simulink library "NCS_Library"  (R2019a)
settings: Solver=VariableStepAuto  StartTime=0.0  StopTime=10.0  RelTol=1e-3
values from neighbouring files (symbols this model uses):
  A = 10    [Parameter.m]
  band = 100000000    [Parameter.m]
  BER = 0    [Parameter.m]
  c = 5000000    [Parameter.m]
  c1 = 4.33    [Parameter.m]
  c2 = 3.16    [Parameter.m]
  CAN2EthernetDelay = 0.000    (= 0)    [Parameter.m]
  cR = 1.5*10^-3    (= 0.0015)    [Parameter.m]
  cw = (cwE * 2 + cwM * (nW_ges-2))/nW_ges    (= 0.1475)    [Parameter.m]
  cwE = 0.35    [Parameter.m]
  cwM = 0.08    [Parameter.m]
  Cycle_Controller = 0    [Parameter.m]
  CyclePLC = 24/1000    (= 0.024)    [Parameter.m]
  d = 800000    [Parameter.m]
  Dr = 0.92    [Parameter.m]
  Ethernet2CANDelay = 0.005    [Parameter.m]
  F_konst = 70892    [Parameter.m]
  FA = 100000    [Parameter.m]
  FB_WB_max = 10000    [Parameter.m]
  FBel_an = iG*nG*F_KZmax*nBan*R_mR/(Dr/2)    (= 28197.4297239)    [Parameter.m]
  FBel_frei = iG*nG*F_KZmax*nBfrei*R_mW/(Dr/2)    (= 29270.6882948)    [Parameter.m]
  Fmaxdyn = 300000    [Parameter.m]
  g = 9.81    [Parameter.m]
  i = 0    [Parameter.m]
  J = 1/2*mA*(Dr/2)^2    (= 158.7)    [Parameter.m]
  k1 = 0.095    [Parameter.m]
  k2 = 9.26/3.6    (= 2.57222222222)    [Parameter.m]
  k3 = 4.63/3.6    (= 1.28611111111)    [Parameter.m]
  mges = 58000    [Parameter.m]
  mu = [mu1 mu2]    [Parameter.m]
  muBel1 = 0.42    [Parameter.m]
  muBel2 = 0.36    [Parameter.m]
  n = 0.001    [Parameter.m]
  n_Mg = 4    [Parameter.m]
  n_WB = 4    [Parameter.m]
  nA = 4    [Parameter.m]
  nBan = 2    [Parameter.m]
  nBfrei = 3    [Parameter.m]
  nM = 4    [Parameter.m]
  nW_an = 4    [Parameter.m]
  P_max = 8200000    [Parameter.m]
  Q = 10    [Parameter.m]
  r_reib = 600    [Parameter.m]
  rho = 1.08    [Parameter.m]
  rhoL = 1.225    [Parameter.m]
  Size = 8    [Parameter.m]
  slip = [s1 s2]    [Parameter.m]
  tol = 0.05    [Parameter.m]
  v00 = 100/3.6    (= 27.7777777778)    [Parameter.m]
  v_grenz = 60/3.6    (= 16.6666666667)    [Parameter.m]
  v_opt = 75/3.6    (= 20.8333333333)    [Parameter.m]
  W_opt = 0.5    [Parameter.m]
  WB = 1    [Parameter.m]
  y_opt = sqrt(W_opt)/((1+sqrt(W_opt))^2+W_opt)    [Parameter.m]
undefined symbols (not defined in the file or in its folder): BUSCapacity, CableLength, controlGate, D_dyn, D_mg, EnableBurst, EnableToF, entity, Entity_out, Gate, Gate_4, Gate_5, Gate_ACK, Gate_copy, Gate_RX, getData, gettime, I_dyn, I_mg, m, magnitude, P_dyn, P_mg, ReadAttributes, readdata, ReadData, ReadSize, sigbuilder_block, Timeout, ToB, ToF, v0, v_d, v_soll
libraries: simulink x176, $bdroot x102
(part 1 of 12)
settings Model: Creator=Moritz  LastModifiedBy=christophunterauer
settings DataIOCC: ReturnWorkspaceOutputs=off
settings DebuggingCC: ArithmeticOperatorsInVariantConditions=warning

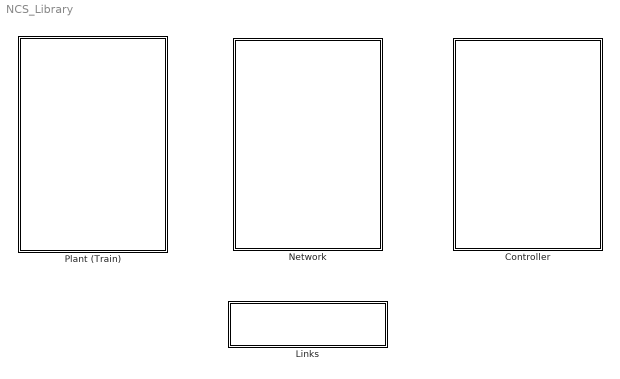
== system NCS_Library ==
  Controller : Subsystem
  Links : Subsystem
  Network : Subsystem
  Plant (Train) : Subsystem

== system NCS_Library/Controller ==
  Controller : Subsystem
      mask Display: disp('Test \n Controller');
  Cookie : Subsystem
  Logic : Subsystem
  Logic with PID : Subsystem
  PID : Subsystem
  PID Controller : Subsystem
      mask Display: disp('PID Controller');
  Subsystem : Subsystem  mask{Scenario=Constant, v_0=0.05, v_d=50}
      mask TypeOptions Scenario: Constant | Arrival | Emergency Break
      mask Callback Scenario:
      | if get_param(gcb,'Scenario') == 1
      |     % acceleration
      |     v0 = 0.05;      % start [m/s]
      |     v_d = 50/3.6;   % desired [m/s]
      | elseif get_param(gcb,'Scenario') == 2
      |     % brake
      |     v0 = 300/3.6;   % start [m/s]
      |     v_d = 300/3.6;  % desired [m/s]
      | end
      mask Callback v_0:
      | if str2double( string(get_param(gcb,'v_0')) ) /3.6 < 0.05*3.6
      |     v0 = 0.05
      | else
      |     v0 = str2double( string(get_param(gcb,'v_0')) ) /3.6;
      | end
      mask Callback v_d: v_d = str2double( string(get_param(gcb,'v_d')) )/3.6;
      mask Display: disp([ 'Scenario Selector' '\n' get_param(gcb,'Scenario') ]);
  Subsystem1 : Subsystem  mask{Scenario=Konstante Fahrt}
      mask TypeOptions Scenario: Konstante Fahrt | Betriebsbremsung | Notbremsung
      mask Display: disp([ 'PID Case' '\n' get_param(gcb,'Scenario') ]);
  Train Controller : Subsystem
      mask Display: disp('Train Controller');
  Train Controller with PID : Subsystem  mask{P_dyn=0.05, I_dyn=0.025, D_dyn=0.001, P_mg=0.05, I_mg=0.025, D_mg=0.001}
      mask Display: disp('Train Controller with PID');

== system NCS_Library/Links ==
  note: Network
  note: Controller
  Mux : Mux  Inputs=3
  tag scope: U=global, Y_M=global, u_1=global, y_M_1=global
  wires:
  Mux/1 -> [y_M_1]
  [u_1] -> ?

== system NCS_Library/Network ==
  Applications : Subsystem
  CAN : Subsystem
  ETB : Subsystem
  Gateway : Subsystem

== system NCS_Library/Plant (Train) ==
  note: Blocks
  note: Modules
  Angetriebene_Achse : Subsystem
  Freie_Achse : Subsystem
  Kupplung : Subsystem
      mask Display: image('Kupplung.png');
  Stellglied : Subsystem
  angetriebener Endwagen : Subsystem
      mask Display: image('Endwagen_angetrieben.png');
  angetriebener Endwagen Merz : Subsystem
      mask Display: image('Endwagen_angetrieben.png');
  angetriebener Mittelwagen : Subsystem
      mask Display: image('Mittlerertriebwagen angetrieben.png');
  angetriebener Wagen : Subsystem
  freier Endwagen : Subsystem
      mask Display: image('Endwagen.png');
  freier Mittelwagen : Subsystem
      mask Display: image('Mittlerertriebwagen.png');
  freier Wagen : Subsystem

== system NCS_Library/Controller/Controller ==
  InFromSensors : Inport
  Delay : Delay  DelayLength=1
  Display : Display
  MATLAB Function1 : MATLAB Function  TreatAsAtomicUnit=on
  OutToActuators : Outport
  wires:
  InFromSensors/1 -> MATLAB Function1/1(Y_M)  "Y_M"
  MATLAB Function1/1(U) -> Display/1, Delay/1
  Delay/1 -> OutToActuators/1

== system NCS_Library/Controller/Cookie ==
  y_M : Inport
  Signal : Inport  Port=2
  Braking Controller : Subsystem
      mask Display: image('seExampleCanController.jpg')
  Bremsstufe : Constant  Value=3
  Constant1 : Constant  Value=0
  Demux : Demux  Outputs=3
  Display : Display
  Display1 : Display
  Display2 : Display
  u : Outport
  wires:
  Demux/3 -> Display/1  "a"
  y_M/1 -> Demux/1
  Constant1/1 -> Braking Controller/3(Notbremse)
  Bremsstufe/1 -> Braking Controller/2(Bremsstufe)
  Demux/2 -> Display2/1, Braking Controller/4(v)  "v"
  Signal/1 -> Braking Controller/1(Fahrstufe)
  Braking Controller/2(fSt) -> Display1/1, u/1  "fSt"

== system NCS_Library/Controller/Logic ==
  y_M : Inport
  Signal : Inport  Port=2
  Braking Controller : Subsystem
      mask Display: image('seExampleCanController.jpg')
  Bremsdauer (Bremsende) : Display
  Bremsdauer (Simulationsende) : Display
  Bremsstufe : Constant  Value=3
  Bremsweg (Bremsende) : Display
  Bremsweg (Simulationsende) : Display
  Constant1 : Constant  Value=0
  Demux : Demux  Outputs=3
  Display : Display
  Display1 : Display
  Display2 : Display
  Scope4 : Scope
  Scope5 : Scope
  Subsystem : Subsystem
  Subsystem1 : Subsystem
  u : Outport
  wires:
  Demux/3 -> Display/1  "a"
  y_M/1 -> Demux/1
  Constant1/1 -> Braking Controller/3(Notbremse)
  Subsystem1/2(Out2) -> Scope5/1, Bremsweg (Bremsende)/1
  Bremsstufe/1 -> Braking Controller/2(Bremsstufe)
  Subsystem/2(Out2) -> Bremsdauer (Bremsende)/1
  Subsystem1/1(Out1) -> Bremsweg (Simulationsende)/1, Scope4/1
  Braking Controller/1(Status) -> Subsystem/1(In1), Subsystem1/1(In1)  "Status"
  Demux/1 -> Subsystem1/2(In2)  "s"
  Demux/2 -> Display2/1, Braking Controller/4(v)  "v"
  Subsystem/1(Out1) -> Bremsdauer (Simulationsende)/1
  Signal/1 -> Braking Controller/1(Fahrstufe)
  Braking Controller/2(fSt) -> Display1/1, u/1  "fSt"

== system NCS_Library/Controller/Logic with PID ==
  y_M : Inport
  Signal : Inport  Port=2
  Demux : Demux  Outputs=3
  Display2 : Display
  Memory : Memory
  Mux : Mux  Inputs=3
  konstante Fahrt : Subsystem
  u : Outport
  wires:
  Signal/1 -> konstante Fahrt/1(Signal)
  y_M/1 -> konstante Fahrt/2(v), Display2/1
  Mux/1 -> u/1
  Demux/3 -> Mux/3  "fSt_WB"
  Demux/2 -> Mux/1  "fSt_pneumatic"
  Demux/1 -> Mux/2  "fSt_dyn"
  konstante Fahrt/1(f_St) -> Memory/1  "fSt"
  Memory/1 -> Demux/1

== system NCS_Library/Controller/PID ==
  y_M : Inport
  Signal : Inport  Port=2
  Add : Sum  Inputs=|+-
  Compare To Zero : simulink/Logic and Bit Operations/Compare To Zero  relop===  OutDataTypeStr=boolean
  Data Type Conversion : DataTypeConversion  OutDataTypeStr=double
  Delay : Delay  DelayLength=1
  Display1 : Display
  Display2 : Display
  Display3 : Display
  Gain1 : Gain  Gain=v_d
  Gain2 : Gain  Gain=-1
  Gain3 : Gain  Gain=-1
  Mux2 : Mux  Inputs=3
  PID Controller2 : simulink/Continuous/PID Controller  Controller=PID  Form=Parallel  TimeDomain=Continuous-time  SampleTime=-1  IntegratorMethod=Forward Euler  FilterMethod=Forward Euler  ControllerParametersSource=internal  P=P_dyn  I=I_dyn  D=D_dyn  UseFilter=on  N=100  TunerSelectOption=Transfer Function Based (PID Tuner App)  InitialConditionSource=internal  InitialConditionForIntegrator=0  InitialConditionForFilter=0  DifferentiatorICPrevScaledInput=0  ExternalReset=none  TrackingMode=off  Kt=1  LimitOutput=on  UpperSaturationLimit=1  LowerSaturationLimit=-1  LinearizeAsGain=on  AntiWindupMode=none  Kb=1  POutMin=[]  POutMax=[]  IOutMin=[]  IOutMax=[]  DOutMin=[]  DOutMax=[]  NOutMin=[]  NOutMax=[]  SumOutMin=[]  SumOutMax=[]  SaturationOutMin=[]  SaturationOutMax=[]  PParamMin=[]  PParamMax=[]  IParamMin=[]  IParamMax=[]  DParamMin=[]  DParamMax=[]  NParamMin=[]  NParamMax=[]  KbParamMin=[]  KbParamMax=[]  KtParamMin=[]  KtParamMax=[]  KbOutMin=[]  KbOutMax=[]  KtOutMin=[]  KtOutMax=[]  IntegratorOutMin=[]  IntegratorOutMax=[]  FilterOutMin=[]  FilterOutMax=[]  SumI1OutMin=[]  SumI1OutMax=[]  SumI2OutMin=[]  SumI2OutMax=[]  SumI3OutMin=[]  SumI3OutMax=[]  SumI4OutMin=[]  SumI4OutMax=[]  SumDOutMin=[]  SumDOutMax=[]  DifferentiatorOutMin=[]  DifferentiatorOutMax=[]  FilterDiffOutCoefMin=[]  FilterDiffOutCoefMax=[]  ReciprocalOutMin=[]  ReciprocalOutMax=[]  SumDenOutMin=[]  SumDenOutMax=[]  SumNumOutMin=[]  SumNumOutMax=[]  DivideOutMin=[]  DivideOutMax=[]  IntegratorContinuousStateAttributes=''  IntegratorStateMustResolveToSignalObject=off  IntegratorRTWStateStorageClass=Auto  FilterContinuousStateAttributes=''  FilterStateMustResolveToSignalObject=off  FilterRTWStateStorageClass=Auto  ParallelPVariant=InternalParameters  IdealPVariant=Disabled  IVariant=InternalParameters  DVariant=InternalParameters  IntegratorVariant=Continuous  SatVariant=Enabled  AWVariant=Passthrough  PCopyVariant=Disabled  TRVariant=Disabled  FdbkBlocksVariant=Forward  IdealPFdbkVariant=Disabled  SatFdbkVariant=Disabled  DerivativeFilterVariant=ContFilter  NVariant=InternalParameters  NCopyVariant=Disabled  FilterICVariant=InternalICsFilter  IntegratorICVariant=InternalICs  ExternalResetVariant=Disabled  TRSumVariant=Passthrough  SumFdbkVariant=Disabled  SumVariant=Sum_PID
  PID Controller3 : simulink/Continuous/PID Controller  Controller=PID  Form=Parallel  TimeDomain=Continuous-time  SampleTime=-1  IntegratorMethod=Forward Euler  FilterMethod=Forward Euler  ControllerParametersSource=internal  P=P_mg  I=I_mg  D=D_mg  UseFilter=on  N=100  TunerSelectOption=Transfer Function Based (PID Tuner App)  InitialConditionSource=internal  InitialConditionForIntegrator=0  InitialConditionForFilter=0  DifferentiatorICPrevScaledInput=0  ExternalReset=none  TrackingMode=off  Kt=1  LimitOutput=on  UpperSaturationLimit=1  LowerSaturationLimit=0  LinearizeAsGain=on  AntiWindupMode=none  Kb=1  POutMin=[]  POutMax=[]  IOutMin=[]  IOutMax=[]  DOutMin=[]  DOutMax=[]  NOutMin=[]  NOutMax=[]  SumOutMin=[]  SumOutMax=[]  SaturationOutMin=[]  SaturationOutMax=[]  PParamMin=[]  PParamMax=[]  IParamMin=[]  IParamMax=[]  DParamMin=[]  DParamMax=[]  NParamMin=[]  NParamMax=[]  KbParamMin=[]  KbParamMax=[]  KtParamMin=[]  KtParamMax=[]  KbOutMin=[]  KbOutMax=[]  KtOutMin=[]  KtOutMax=[]  IntegratorOutMin=[]  IntegratorOutMax=[]  FilterOutMin=[]  FilterOutMax=[]  SumI1OutMin=[]  SumI1OutMax=[]  SumI2OutMin=[]  SumI2OutMax=[]  SumI3OutMin=[]  SumI3OutMax=[]  SumI4OutMin=[]  SumI4OutMax=[]  SumDOutMin=[]  SumDOutMax=[]  DifferentiatorOutMin=[]  DifferentiatorOutMax=[]  FilterDiffOutCoefMin=[]  FilterDiffOutCoefMax=[]  ReciprocalOutMin=[]  ReciprocalOutMax=[]  SumDenOutMin=[]  SumDenOutMax=[]  SumNumOutMin=[]  SumNumOutMax=[]  DivideOutMin=[]  DivideOutMax=[]  IntegratorContinuousStateAttributes=''  IntegratorStateMustResolveToSignalObject=off  IntegratorRTWStateStorageClass=Auto  FilterContinuousStateAttributes=''  FilterStateMustResolveToSignalObject=off  FilterRTWStateStorageClass=Auto  ParallelPVariant=InternalParameters  IdealPVariant=Disabled  IVariant=InternalParameters  DVariant=InternalParameters  IntegratorVariant=Continuous  SatVariant=Enabled  AWVariant=Passthrough  PCopyVariant=Disabled  TRVariant=Disabled  FdbkBlocksVariant=Forward  IdealPFdbkVariant=Disabled  SatFdbkVariant=Disabled  DerivativeFilterVariant=ContFilter  NVariant=InternalParameters  NCopyVariant=Disabled  FilterICVariant=InternalICsFilter  IntegratorICVariant=InternalICs  ExternalResetVariant=Disabled  TRSumVariant=Passthrough  SumFdbkVariant=Disabled  SumVariant=Sum_PID
  Signal1 : InportShadow  Port=2
  Transport Delay : TransportDelay  Commented=on  DelayTime=Cycle_Controller
  u : Outport
  wires:
  Add/1 -> Gain2/1, Gain3/1, Display3/1  "e"
  y_M/1 -> Add/2  "y_m"
  Gain1/1 -> Add/1  "w"
  Signal/1 -> Display2/1, Gain1/1
  Signal1/1 -> Compare To Zero/1
  Mux2/1 -> Delay/1, Display1/1  "f_St"
  Gain2/1 -> PID Controller3/1
  Gain3/1 -> PID Controller2/1  "f_St,dyn"
  Compare To Zero/1 -> Data Type Conversion/1
  Data Type Conversion/1 -> Mux2/1  "f_St,pneumatic"
  PID Controller2/1 -> Mux2/2  "f_St,dyn"
  PID Controller3/1 -> Mux2/3  "f_St,mg"
  Delay/1 -> u/1

== system NCS_Library/Controller/PID Controller ==
  InFromNetwork : Inport
  Signal1 : Inport  Port=2
  Demux : Demux
  Mux : Mux
  PID{,1..3} (4 alike) : $bdroot/Controller/PID  SystemSampleTime=-1
  Signal2 : InportShadow  Port=2
  Signal3 : InportShadow  Port=2
  Signal4 : InportShadow  Port=2
  Transport Delay : TransportDelay  DelayTime=CyclePLC
  OutToController : Outport
  wires:
  InFromNetwork/1 -> Demux/1  "Y_M"
  Mux/1 -> Transport Delay/1  "U"
  PID/1 -> Mux/1  "u_1"
  PID1/1 -> Mux/2  "u_2"
  PID2/1 -> Mux/3  "u_3"
  PID3/1 -> Mux/4  "u_4"
  Demux/1 -> PID/1  "y_M_1"
  Demux/2 -> PID1/1  "y_M_2"
  Demux/3 -> PID2/1  "y_M_3"
  Demux/4 -> PID3/1  "y_M_4"
  Signal1/1 -> PID/2
  Signal2/1 -> PID1/2
  Signal3/1 -> PID2/2
  Signal4/1 -> PID3/2
  Transport Delay/1 -> OutToController/1

== system NCS_Library/Controller/Subsystem ==
  Constant : Constant  Value=Scenario
  Multiport Switch : MultiPortSwitch
  Signal Builder : Subsystem  Tag=STV Subsys  LoadFcn=sigbuilder_block('load');  StartFcn=sigbuilder_block('start');  StopFcn=sigbuilder_block('stop');  ClipboardFcn=sigbuilder_block('clipboard');  mask(Sigbuilder block){tuvar=[0:10]}
      mask help: Simulink:masks:SigbuilderBlock_MD
      mask init:
      | if ~strcmp(get_param(bdroot(gcbh),'SimulationStatus'),'stopped') tuvar = sigbuilder_block('maskInit'); end
      settings: CopyFcn=sigbuilder_block('copy');  DeleteFcn=sigbuilder_block('delete');  ModelCloseFcn=sigbuilder_block('modelClose');  PreSaveFcn=sigbuilder_block('preSave');  PauseFcn=sigbuilder_block('pause');  ContinueFcn=sigbuilder_block('continue');  NameChangeFcn=sigbuilder_block('namechange');  OpenFcn=sigbuilder_block('open',[643.5 127.5 500.25 477 ]);  CloseFcn=sigbuilder_block('close');
      mask Display: plot(0, 0, 100, 100,[2, 2, 32, 32, 2], [68, 8, 8, 68, 68],[32, 2], [38, 38], [32, 19, 2],[53, 60, 44], [32, 17, 17, 2],[16, 16, 31, 31]);txt = getActiveGroup(gcbh);text(2, 100, txt,'verticalAlignment', 'top');
  Signal : Outport
  wires:
  Signal Builder/2(Arrival) -> Multiport Switch/3
  Signal Builder/1(Constant) -> Multiport Switch/2
  Signal Builder/3(Notbremsung) -> Multiport Switch/4
  Constant/1 -> Multiport Switch/1
  Multiport Switch/1 -> Signal/1

== system NCS_Library/Controller/Subsystem1 ==
  Constant : Constant  Value=Scenario
  Multiport Switch : MultiPortSwitch
  Signal Builder : Subsystem  Tag=STV Subsys  LoadFcn=sigbuilder_block('load');  StartFcn=sigbuilder_block('start');  StopFcn=sigbuilder_block('stop');  ClipboardFcn=sigbuilder_block('clipboard');  mask(Sigbuilder block){tuvar=[0:10]}
      mask help: Simulink:masks:SigbuilderBlock_MD
      mask init:
      | if ~strcmp(get_param(bdroot(gcbh),'SimulationStatus'),'stopped') tuvar = sigbuilder_block('maskInit'); end
      settings: CopyFcn=sigbuilder_block('copy');  DeleteFcn=sigbuilder_block('delete');  ModelCloseFcn=sigbuilder_block('modelClose');  PreSaveFcn=sigbuilder_block('preSave');  PauseFcn=sigbuilder_block('pause');  ContinueFcn=sigbuilder_block('continue');  NameChangeFcn=sigbuilder_block('namechange');  OpenFcn=sigbuilder_block('open',[726 36 708 711 ]);  CloseFcn=sigbuilder_block('close');
      mask Display: plot(0, 0, 100, 100,[2, 2, 32, 32, 2], [68, 8, 8, 68, 68],[32, 2], [38, 38], [32, 19, 2],[53, 60, 44], [32, 17, 17, 2],[16, 16, 31, 31]);txt = getActiveGroup(gcbh);text(2, 100, txt,'verticalAlignment', 'top');
  Signal : Outport
  wires:
  Multiport Switch/1 -> Signal/1
  Constant/1 -> Multiport Switch/1
  Signal Builder/3(Notbremsung) -> Multiport Switch/4
  Signal Builder/1(Konstante Fahrt) -> Multiport Switch/2
  Signal Builder/2(Betriebsbremsung) -> Multiport Switch/3

== system NCS_Library/Controller/Train Controller ==
  InFromNetwork : Inport
  Signal1 : Inport  Port=2
  Demux : Demux
  Logic{,1..3} (4 alike) : $bdroot/Controller/Logic  SystemSampleTime=-1
  Mux : Mux
  Signal2 : InportShadow  Port=2
  Signal3 : InportShadow  Port=2
  Signal4 : InportShadow  Port=2
  OutToController : Outport
  wires:
  InFromNetwork/1 -> Demux/1  "Y_M"
  Mux/1 -> OutToController/1  "U"
  Logic/1 -> Mux/1  "u_1"
  Logic1/1 -> Mux/2  "u_2"
  Logic2/1 -> Mux/3  "u_3"
  Logic3/1 -> Mux/4  "u_4"
  Demux/1 -> Logic/1  "y_M_1"
  Demux/2 -> Logic1/1  "y_M_2"
  Demux/3 -> Logic2/1  "y_M_3"
  Demux/4 -> Logic3/1  "y_M_4"
  Signal1/1 -> Logic/2
  Signal2/1 -> Logic1/2
  Signal3/1 -> Logic2/2
  Signal4/1 -> Logic3/2

== system NCS_Library/Controller/Train Controller with PID ==
  InFromNetwork : Inport
  Signal1 : Inport  Port=2
  Display : Display
  MATLAB Function : MATLAB Function  TreatAsAtomicUnit=on
  MATLAB Function1 : MATLAB Function  TreatAsAtomicUnit=on
  PID : $bdroot/Controller/PID  SystemSampleTime=-1
  OutToController : Outport  PortDimensions=[3 20]
  wires:
  Signal1/1 -> PID/2
  InFromNetwork/1 -> Display/1, MATLAB Function/1(Y_M)  "Y_M"
  PID/1 -> MATLAB Function1/1(u)
  MATLAB Function1/1(U) -> OutToController/1
  MATLAB Function/1(v) -> PID/1

== system NCS_Library/Network/Applications ==
  Failure Control : Subsystem
  Failure Control CAN : Subsystem
  Multiplexer : Subsystem
  NetworkSelector : Subsystem  mask{NetworkType=Reference, band=10 MB/s, BER=0.01, RD=50.0}
      mask prompts: NetworkType "Network Type"; band "Bandwidth"; BER "Bit Error Rate [%]"; RD "Delay Reference Network [ms]"
      mask help: It is recomended to comment out the unused networks!
      mask TypeOptions NetworkType: Reference | EthernetCAN | Ethernet | EthernetCAN_Ring
      mask TypeOptions band: 10 MB/s | 100 MB/s | 1 GB/s
      mask Callback band:
      | bandwidth = get_param(gcb,'band');
      | 
      | switch bandwidth
      |     case '10 MB/s'
      |         band = 10^7;
      |     case '100 MB/s'
      |         band = 10^8;
      |     case '1 GB/s'
      |         band = 10^9;
      |     otherwise
      |         band = 1;
      | end
      | clear bandwidth
      mask Callback BER: BER = get_param(gcb,'BER') / 100;
      mask Callback RD:
      | % convert delay from char to string and from string to num
      | % no idea, why it is saved as char first
      | ReferenceDelay = str2double( string(get_param(gcb,'RD')) ) / 1000;
      mask DialogControl Container3 Prompt: Ethernet Parameters
      mask Display: disp([ 'NetworkSelector' '\n' '\n' get_param(gcb,'NetworkType') ]);
  Subsystem : Subsystem
  TRDP Timeout : Subsystem
  Watch Dog : Subsystem

== system NCS_Library/Network/CAN ==
  note: CAN 2
  note: CAN 1
  CAN BUS : Subsystem  mask{BusID=1, Capacity=500000, LossRate=0.001}
      mask prompts: Capacity "Channel capacity(bit/s)"; LossRate "Loss probability(0-1)"
      mask help: Simulate a CAN Bus
      mask init:
      | % global BUSCapacity;
      | BUSCapacity = Capacity;
      mask Callback Capacity: evalin('base',['BUSCapacity=' num2str(get_param(gcb,'Capacity')) ';']);
      mask Display: disp(['CAN Bus ' get_param(gcb,'BusID')]);
  CAN BUS1 : Subsystem  mask{BusID=2, Capacity=500000, LossRate=0.001}
      mask prompts: Capacity "Channel capacity(bit/s)"; LossRate "Loss probability(0-1)"
      mask help: Simulate a CAN Bus
      mask init:
      | % global BUSCapacity;
      | BUSCapacity = Capacity;
      mask Callback Capacity: evalin('base',['BUSCapacity=' num2str(get_param(gcb,'Capacity')) ';']);
      mask Display: disp(['CAN Bus ' get_param(gcb,'BusID')]);
  CAN Node 1 : Subsystem  mask(CAN Node){MsgID=1, IDRange=[1:25], T_Tx=0, SensorType=Velocity, MsgSize=8, IDSubscription=[0,0,0,0,0,0,0,0,0,0,0,0,0,0,0,0,0,0,0,0,0,0,0,0,0], EnableToF=off, ToF=0}
      mask prompts: MsgID "CAN identifier (ID)"; IDRange "Range of all IDs"; SensorType "Type"; MsgSize "Data size (0-8 bytes)"; IDSubscription "IDs of messages subscribed to accept (0-no, 1-yes)"; EnableToF "Failure"; ToF "Time of Failure [s]"
      mask help: CAN Node transmits and receives messages over the CANbus.
      mask init:
      | if SensorType > 3
      |     T_Tx = inf;
      | end
      mask TypeOptions SensorType: Position Sensor | Velocity Sensor | Acceleration Sensor | Actuator
      mask Callback EnableToF:
      | % Control parameter visiblity
      | % Disable Tx dialog, if it is not needed, because of a passive ED,
      | % which only receives.
      | 
      | % Get value
      | ToF = get_param(gcb,'EnableToF');
      | % ToB = get_param(gcb,'EnableBurst');
      | 
      | 
      | % Set the 'MaskVisibilities' property for each box
      | 
      | On = {'on','on','on','on','on','on','on','on'}; % Init
      | 
      | % Disable Tx Dialog, if not needed
      | if strcmp('off',ToF)
      |     On{8} = 'off';
      | end
      | 
      | set_param(gcb,'MaskEnables',On );
      mask DialogControl Container3 Prompt: Interrupts
      mask Display: disp(['CAN ID:' get_param(gcb,'MsgID')]);
  CAN Node 2 : Subsystem  mask(CAN Node){MsgID=1, IDRange=[1:25], T_Tx=0, SensorType=Velocity, MsgSize=8, IDSubscription=[0,0,0,0,0,0,0,0,0,0,0,0,0,0,0,0,0,0,0,0,0,0,0,0,0], EnableToF=off, ToF=0}
      mask prompts: MsgID "CAN identifier (ID)"; IDRange "Range of all IDs"; SensorType "Type"; MsgSize "Data size (0-8 bytes)"; IDSubscription "IDs of messages subscribed to accept (0-no, 1-yes)"; EnableToF "Failure"; ToF "Time of Failure [s]"
      mask help: CAN Node transmits and receives messages over the CANbus.
      mask init:
      | if SensorType > 3
      |     T_Tx = inf;
      | end
      mask TypeOptions SensorType: Position Sensor | Velocity Sensor | Acceleration Sensor | Actuator
      mask Callback EnableToF:
      | % Control parameter visiblity
      | % Disable Tx dialog, if it is not needed, because of a passive ED,
      | % which only receives.
      | 
      | % Get value
      | ToF = get_param(gcb,'EnableToF');
      | % ToB = get_param(gcb,'EnableBurst');
      | 
      | 
      | % Set the 'MaskVisibilities' property for each box
      | 
      | On = {'on','on','on','on','on','on','on','on'}; % Init
      | 
      | % Disable Tx Dialog, if not needed
      | if strcmp('off',ToF)
      |     On{8} = 'off';
      | end
      | 
      | set_param(gcb,'MaskEnables',On );
      mask DialogControl Container3 Prompt: Interrupts
      mask Display: disp(['CAN ID:' get_param(gcb,'MsgID')]);
  CAN Node 3 : Subsystem  mask(Gateway Transceiver){FromBus_number=2, ToBus_number=1, MsgSize=8, IDSubscription=[0,0,0,0,0,0,0,1,1,1,1,1,1,1,1,1,1,0,0,0,0,0,0,0,0,0], IDRange=[0:25], Takt=0.100, Offset=0, ideal=on}
      mask prompts: FromBus_number "From Bus"; ToBus_number "To Bus"; MsgSize "Data size (0-8 bytes)"; IDSubscription "IDs of messages subscribed to accept (0-no, 1-yes)"; IDRange "Range of all IDs"; Takt "Takt [ms]"; Offset "Offset [ms]"; ideal "Ideal Behavior"
      mask help: Gateway Transceiver transmits and receives messages over the CANbus.
      mask init:
      | s_from = num2str(FromBus_number);
      | s_to = num2str(ToBus_number);
      | 
      | RX_Bus = strcat('FromBus_',s_from);
      | ACK_Bus = strcat('FromBus_',s_to);
      | TX_Bus = strcat('ToBus_',s_to);
      | 
      | mask_path = getfullname(gcb);
      | send_path = strcat(mask_path,'/TX Message');
      | receive_path = strcat(mask_path,'/RX Message');
      | ack_path = strcat(mask_path,'/ACK Message');
      | 
      | set_param(send_path,'Multicasttag',TX_Bus);
      | set_param(receive_path,'Multicasttag',RX_Bus);
      | set_param(ack_path,'Multicasttag',ACK_Bus);
      mask Display: disp(['Gateway\nBus ' get_param(gcb,'FromBus_number') ' to Bus ' get_param(gcb,'ToBus_number')]);
  CAN Node 4 : Subsystem  mask(Gateway Transceiver){FromBus_number=1, ToBus_number=2, MsgSize=8, IDSubscription=[0,1,1,1,1,1,1,0,0,0,0,0,0,0,0,0,0,0,0,0,0,0,0,1,1,1], IDRange=[0:25], Takt=0.100, Offset=0, ideal=on}
      mask prompts: FromBus_number "From Bus"; ToBus_number "To Bus"; MsgSize "Data size (0-8 bytes)"; IDSubscription "IDs of messages subscribed to accept (0-no, 1-yes)"; IDRange "Range of all IDs"; Takt "Takt [ms]"; Offset "Offset [ms]"; ideal "Ideal Behavior"
      mask help: Gateway Transceiver transmits and receives messages over the CANbus.
      mask init: same as NCS_Library/Network/CAN/CAN Node 3
      mask Display: disp(['Gateway\nBus ' get_param(gcb,'FromBus_number') ' to Bus ' get_param(gcb,'ToBus_number')]);
  Logik : Subsystem  mask{Takt_fast=0.085, Takt_slow=0.100, Takt_wait=0.1, Offset=0, Delay_input=0.01, Copy_on=off, Wait_on=off}
      mask prompts: Takt_fast "Takt of fast Network [ms]"; Takt_slow "Takt of slow Network [ms]"; Takt_wait "Takt to downsample [ms]"; Offset "Offset [ms]"; Delay_input "Processing Delay [ms]"; Copy_on "Activate Upsampling"; Wait_on "Activate Downsampling"
      mask init:
      | Delay = Delay_input - 0.001;
      | 
      | Wait_off = ~Wait_on;
  wires:
  Logik/2(Out_fast) -> CAN Node 3/1(Entity_transmit)
  Logik/1(Out_slow) -> CAN Node 4/1(Entity_transmit)
  CAN Node 4/1(Entity_received) -> Logik/1(In_fast)
  CAN Node 3/1(Entity_received) -> Logik/2(In_slow)
